simulink model "sgMdl_IO3xx_Interrupt_modelTrigger"  (R2024b)
settings: Solver=FixedStepAuto  StartTime=0.0  StopTime=inf  RelTol=1e-3  EnableMultiTasking=on
undefined symbols (not defined in the file): Pull, pull, up
libraries: speedgoatlib_fpga_inta x1, simulink x1, speedgoatlib_interrupt x1, speedgoatlib_fpga x1
Description:
  | IO3xx Interrupt - Model Trigger
settings Model: ModifiedByFormat=Speedgoat  SimulationMode=external  ExtModeTrigDuration=100000  Creator=Speedgoat  LastModifiedBy=Speedgoat
settings SolverCC: ConcurrentTasks=on  AlgebraicLoopSolver=TrustRegion  PositivePriorityOrder=on  InsertRTBMode=Never (minimum delay)
settings DataIOCC: SaveFormat=Array  SaveState=on  SignalLoggingName=logsOut
settings OptimizationCC: BlockReduction=off  BooleanDataType=off  OptimizeBlockIOStorage=off  BufferReuse=off  GlobalBufferReuse=off  ExpressionFolding=off  LocalBlockOutputs=off  InitFltsAndDblsToZero=on  OptimizeDataStoreBuffers=off  BusAssignmentInplaceUpdate=off
settings DebuggingCC: SaveWithParameterizedLinksMsg=none  UnderspecifiedInitializationDetection=Classic  MergeDetectMultiDrivingBlocksExec=none  CheckExecutionContextPreStartOutputMsg=on  SignalResolutionControl=TryResolveAllWithWarning  TasksWithSamePriorityMsg=none  UnconnectedInputMsg=warning  UnconnectedOutputMsg=warning  UnconnectedLineMsg=warning  SFUnexpectedBacktrackingDiag=warning  SFNoUnconditionalDefaultTransitionDiag=warning  SFExecutionAtInitializationDiag=none  ArithmeticOperatorsInVariantConditions=warning
settings HardwareCC: ProdBitPerLong=64  ProdLongLongMode=on  ProdHWDeviceType=Intel->x86-64 (Linux 64)
settings ModelReferenceCC: EnableRefExpFcnMdlSchedulingChecks=on  PropagateSignalLabelsOutOfModel=off
settings SFSimCC: SimUseLocalCustomCode=off  SimTargetLang=C++
settings RTWCC: Description=Speedgoat Real-Time Target Machine  SystemTargetFile=speedgoat.tlc  TemplateMakefile=slrealtime_default_tmf  PostCodeGenCommand=sg.model.build.makeCfg(bdroot, buildInfo);  RTWUseLocalCustomCode=off  Toolchain=Simulink Real-Time Toolchain  BuildConfiguration=Faster Runs  TargetLang=C++  GPUComputeCapability=3.5  DLArmComputeVersion=19.05
settings CodeAppCC: StateflowObjectComments=on
settings SimulinkRealTimeTargetCC: SubcomponentCodeInterfacePackaging=Reusable function  MATLABClassNameForMDSCustomization=Simulink.SoftwareTarget.GRTCustomization  InstructionSetFMA=off  LogToMDFFile=off  SLRTFileLogMaxRuns=10  UseGCCFastMath=on
settings ConfigComp: CovMetricSettings=dw  CovSaveCumulativeToWorkspaceVar=on  CovSaveSingleToWorkspaceVar=on  CovExternalEMLEnable=off  CovSFcnEnable=off  CovBoundaryAbsTol=1.0e-5

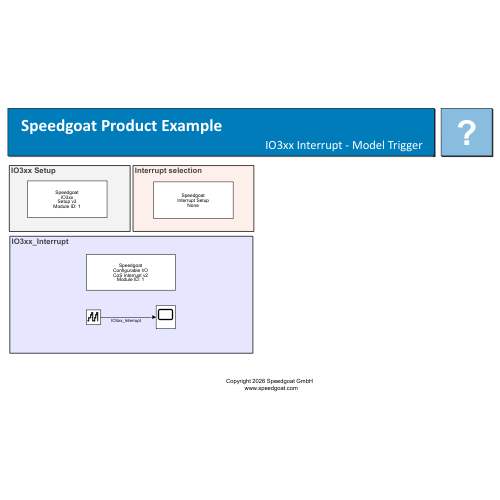
[thumbnail: Simulink's stored preview of the top-level diagram]
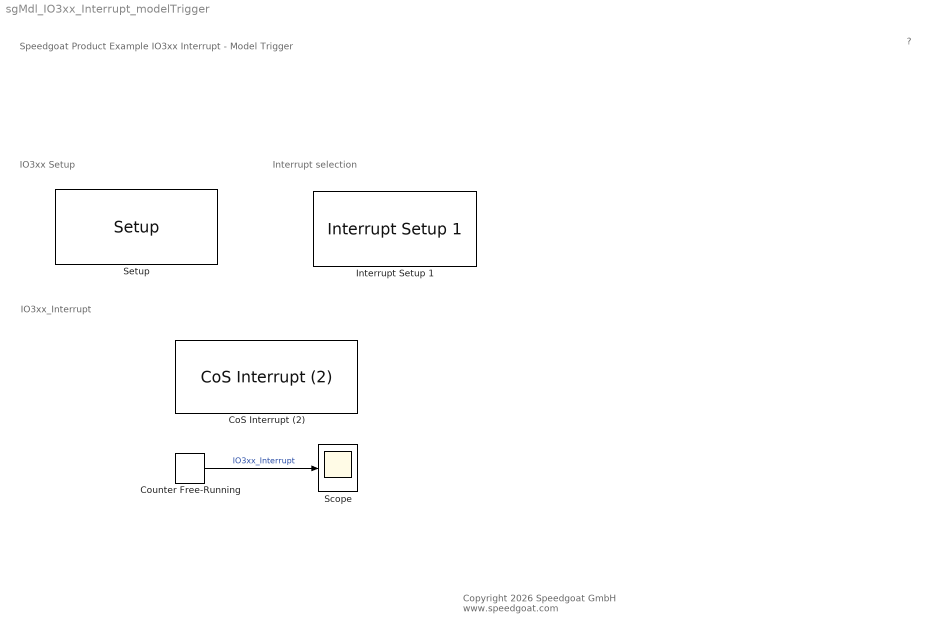
== system sgMdl_IO3xx_Interrupt_modelTrigger ==
  note: Interrupt selection
  note: IO3xx_Interrupt
  note: IO3xx Setup
  note: Speedgoat Product Example
      | IO3xx Interrupt - Model Trigger
  note: ?
  note: Copyright 2026 Speedgoat GmbH
      |  www.speedgoat.com
  CoS Interrupt (2) : speedgoatlib_fpga_inta/CoS Interrupt (2)  id=1  channel=[1]  ts=0.001  fpga_frequency=0  int_source=internally generated  mode=0  debounce=500e-4  delay=0  ad_settings=off  division=0  multiplication=0  gap=1e-3  int_freq=1e3  freq_2_time=1.00000e-03  event=off  timestamp=off  flag=off
      settings: SourceProductName=Interrupt
  Counter Free-Running : simulink/Sources/Counter Free-Running  NumBits=32  tsamp=0.001
  Interrupt Setup 1 : speedgoatlib_interrupt/Interrupt Setup 1  parModuleTrigger=on  parPollingMode=off  parPriorityConf=High  parPriority=90  confStartFcn=IO317_100k_v2_start_public  confStopFcn=IO317_100k_v2_stop_public  confIsrFcn=IO317_100k_v2_isr_public  confMapFcn=IO317_100k_v2_map_public  confHookFile=io317_100k_v2_int_hooks.c  confIrqNr=-1  confIsPolling=off  confModID=33554177  confSelectedInt=None  confSelectedId=[]  confSelectedChannel=[]  confData=[90 1]  confForcePollingMode=off
  Scope : Scope
  Setup : speedgoatlib_fpga/Setup/Setup  board=Please select...  id=1  pciSlot=-1  device_id=1  bitstreamFilePath=C:\SVN\speedgoatlib\releases\10.0.0\product_examples\IO3xx_Interrupt  bitstreamFile=Please select...  fpgaFreq=[75000000 100000000]  enableDma=off  rearEnb_1=off  rearIO_1=None  rearEnb_2=off  rearIO_2=None  ProgSpiFlash=off  ProgBPIFlash=off  useFpgaDmaController=off  dmaTrigDropdown=Model Step  dmaTrigSelect=0  dmaStopOnOverload=on  dmaModeSequential=on  dmaModeParallel=off  PullRPort15=pull-up 3.3V  PullRPort31=pull-up 3.3V  PullRPort47=pull-up 3.3V  PullRPort63=pull-up 3.3V  diffLineTermination_1=on  diffLineTermination_2=on  diffLineTermination_3=on  diffLineTermination_4=on  diffLineTermination_5=on  diffLineTermination_6=on  diffLineTermination_7=on  diffLineTermination_8=on  diffLineTermination_9=on  diffLineTermination_10=on  diffLineTermination_11=on  diffLineTermination_12=on  diffLineTermination_13=on  diffLineTermination_14=on  diffLineTermination_15=on  diffLineTermination_16=on  diffLineTermination_17=on  diffLineTermination_18=on  diffLineTermination_19=on  diffLineTermination_20=on  diffLineTermination_21=on  diffLineTermination_22=on  diffLineTermination_23=on  diffLineTermination_24=on  diffLineTermination_25=on  diffLineTermination_26=on  diffLineTermination_27=on  diffLineTermination_28=on  diffLineTermination_29=on  diffLineTermination_30=on  diffLineTermination_31=on  diffLineTermination_32=on  ioVoltageDropDown1=3.3V  pullResistorDropDown1_1=Pull-up  pullResistorDropDown1_2=Pull-up  pullResistorDropDown1_3=Pull-up  pullResistorDropDown1_4=Pull-up  pullResistorDropDown1_5=Pull-up  pullResistorDropDown1_6=Pull-up  pullResistorDropDown1_7=Pull-up  pullResistorDropDown1_8=Pull-up  ttlIsImplementedCheckBox1=off  pullResistorDropDown2=Pull-up  ioVoltageDropDown2=3.3V  ttlIsImplementedCheckBox2=off  pullResistorDropDown3=Pull-up  ioVoltageDropDown3=3.3V  ttlIsImplementedCheckBox3=off  pullResistorDropDown4=Pull-up  ioVoltageDropDown4=3.3V  ttlIsImplementedCheckBox4=off  pullResistorDropDown5=Pull-up  ioVoltageDropDown5=3.3V  ttlIsImplementedCheckBox5=off  pullResistorDropDown6=Pull-up  ioVoltageDropDown6=3.3V  ttlIsImplementedCheckBox6=off  pullResistorDropDown7=Pull-up  ioVoltageDropDown7=3.3V  ttlIsImplementedCheckBox7=off  pullResistorDropDown8=Pull-up  ioVoltageDropDown8=3.3V  ttlIsImplementedCheckBox8=off  terminationCheckBox1=off  terminationCheckBox2=off  terminationCheckBox3=off  terminationCheckBox4=off  diffIsImplementedCheckBox1=off  terminationCheckBox5=off  terminationCheckBox6=off  terminationCheckBox7=off  terminationCheckBox8=off  diffIsImplementedCheckBox2=off  terminationCheckBox9=off  terminationCheckBox10=off  terminationCheckBox11=off  terminationCheckBox12=off  diffIsImplementedCheckBox3=off  terminationCheckBox13=off  terminationCheckBox14=off  terminationCheckBox15=off  terminationCheckBox16=off  diffIsImplementedCheckBox4=off  terminationCheckBox17=off  terminationCheckBox18=off  terminationCheckBox19=off  terminationCheckBox20=off  diffIsImplementedCheckBox5=off  terminationCheckBox21=off  terminationCheckBox22=off  terminationCheckBox23=off  terminationCheckBox24=off  diffIsImplementedCheckBox6=off  terminationCheckBox25=off  terminationCheckBox26=off  terminationCheckBox27=off  terminationCheckBox28=off  diffIsImplementedCheckBox7=off  terminationCheckBox29=off  terminationCheckBox30=off  terminationCheckBox31=off  terminationCheckBox32=off  diffIsImplementedCheckBox8=off  PullRPort0_1=pull-up  VioPort0_1=3.3V  PullRPort1_1=pull-up  VioPort1_1=3.3V  PullRPort2_1=pull-up  VioPort2_1=3.3V  PullRPort3_1=pull-up  VioPort3_1=3.3V  PullRPort4_1=pull-up  VioPort4_1=3.3V  PullRPort5_1=pull-up  VioPort5_1=3.3V  PullRPort6_1=pull-up  VioPort6_1=3.3V  diffLineTermination_rear1_1=on  diffLineTermination_rear1_2=on  diffLineTermination_rear1_3=on  diffLineTermination_rear1_4=on  diffLineTermination_rear1_5=on  diffLineTermination_rear1_6=on  diffLineTermination_rear1_7=on  diffLineTermination_rear1_8=on  PullRPort0_2=pull-up  VioPort0_2=3.3V  PullRPort1_2=pull-up  VioPort1_2=3.3V  PullRPort2_2=pull-up  VioPort2_2=3.3V  PullRPort3_2=pull-up  VioPort3_2=3.3V  PullRPort4_2=pull-up  VioPort4_2=3.3V  PullRPort5_2=pull-up  VioPort5_2=3.3V  PullRPort6_2=pull-up  VioPort6_2=3.3V  diffLineTermination_rear2_1=on  diffLineTermination_rear2_2=on  diffLineTermination_rear2_3=on  diffLineTermination_rear2_4=on  diffLineTermination_rear2_5=on  diffLineTermination_rear2_6=on  diffLineTermination_rear2_7=on  diffLineTermination_rear2_8=on
      settings: SourceProductName=IO3xx
  wires:
  Counter Free-Running/1 -> Scope/1  "IO3xx_Interrupt"
